simulink model "double_tank_system"  (R2020b)
settings: Solver=VariableStepAuto  StartTime=0.0  StopTime=10.0  RelTol=1e-3
values from neighbouring files (symbols this model uses):
  A1 = 1    [init_double_tank_system.m]
  A2 = 1    [init_double_tank_system.m]
  Ar = 0.1    [init_double_tank_system.m]
  g = 9.81    [init_double_tank_system.m]
  H1 = 10    [init_double_tank_system.m]
  H2 = 0    [init_double_tank_system.m]
settings Model: Creator=root  LastModifiedBy=root

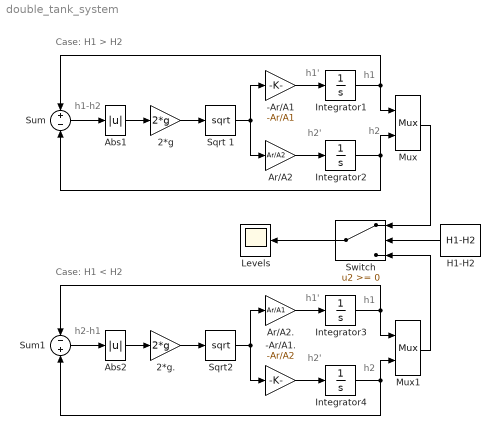
== system double_tank_system ==
  note: h1'
  note: h2-h1
  note: h2'
  note: Case: H1 > H2
  note: Case: H1 < H2
  note: h2'
  note: h1
  note: h2
  note: h1
  note: h1-h2
  note: h2
  note: h1'
  -Ar/A1 : Gain  Gain=-Ar/A1
  -Ar/A1. : Gain  Gain=-Ar/A2
  2*g : Gain  Gain=2*g
  2*g. : Gain  Gain=2*g
  Abs1 : Abs
  Abs2 : Abs
  Ar/A2 : Gain  Gain=Ar/A2
  Ar/A2. : Gain  Gain=Ar/A1
  H1-H2 : Constant  Value=H1-H2
  Integrator1 : Integrator  InitialCondition=H1
  Integrator2 : Integrator  InitialCondition=H2
  Integrator3 : Integrator  InitialCondition=H1
  Integrator4 : Integrator  InitialCondition=H2
  Levels : Scope
  Mux : Mux  Inputs=2
  Mux1 : Mux  Inputs=2
  Sqrt 1 : Sqrt  SaturateOnIntegerOverflow=on
  Sqrt2 : Sqrt  SaturateOnIntegerOverflow=on
  Sum : Sum  Inputs=+-
  Sum1 : Sum  Inputs=-+
  Switch : Switch
  wires:
  Integrator3/1 -> Mux1/1, Sum1/1
  Mux1/1 -> Switch/3
  Mux/1 -> Switch/1
  Abs1/1 -> 2*g/1
  -Ar/A1./1 -> Integrator4/1
  Integrator2/1 -> Sum/2, Mux/2
  2*g/1 -> Sqrt 1/1
  Integrator4/1 -> Mux1/2, Sum1/2
  Integrator1/1 -> Mux/1, Sum/1
  Sum/1 -> Abs1/1
  H1-H2/1 -> Switch/2
  Ar/A2/1 -> Integrator2/1
  -Ar/A1/1 -> Integrator1/1
  Ar/A2./1 -> Integrator3/1
  Sqrt 1/1 -> Ar/A2/1, -Ar/A1/1
  Abs2/1 -> 2*g./1
  Sum1/1 -> Abs2/1
  Switch/1 -> Levels/1
  Sqrt2/1 -> Ar/A2./1, -Ar/A1./1
  2*g./1 -> Sqrt2/1
